simulink model "halfcontcon"  (R2021a)
settings: Solver=VariableStepAuto  StartTime=0.0  StopTime=5  FixedStep=1e-6  RelTol=1e-3
values from neighbouring files (symbols this model uses):
  Tr = (Pr*746)/(wr)    (= 20.3536435794)    [halfcontrolledconverter.m]
  vcontrol = cosd(alpha)    [halfcontrolledconverter.m]
  Vm = Vs_rms*(2)^(0.5)    (= 325.269119346)    [halfcontrolledconverter.m]
libraries: spsDiodeLib x6, spsVoltageMeasurementLib x3, spsCurrentMeasurementLib x2, simulink_extras x2, spsMonostableLib x2, spsThyristorLib x2, spsACVoltageSourceLib x1, spsDCMachineLib x1, spsGroundLib x1, spsSeriesRLCBranchLib x1, spspowerguiLib x1
settings Model: Creator=dinesh  LastModifiedBy=mluser
settings SolverCC: ZeroCrossAlgorithm=Adaptive  AlgebraicLoopSolver=TrustRegion
settings DataIOCC: ReturnWorkspaceOutputs=off
settings DebuggingCC: IgnoredZcDiagnostic=none  SFMachineParentedDataDiag=warning  ArithmeticOperatorsInVariantConditions=warning
settings SFSimCC: SimUseLocalCustomCode=off  CustomCodeUndefinedFunction=UseInterfaceOnly
settings RTWCC: RTWUseLocalCustomCode=off

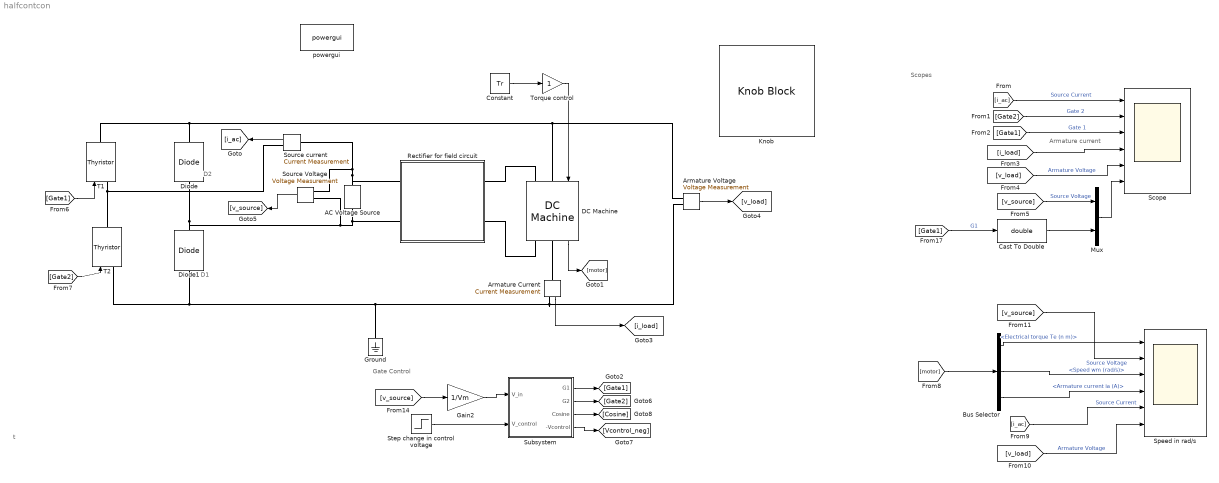
== system halfcontcon ==
  note: Armature current
  note: D2
  note: D1
  note: t
  note: Scopes
  note: Gate Control
  AC Voltage Source : spsACVoltageSourceLib/AC Voltage Source  Amplitude=Vm  Phase=0  Frequency=50  SampleTime=0  Measurements=None  BusType=swing  Pref=10e3  Qref=0  Qmin=-inf  Qmax=+inf
  Armature Current : spsCurrentMeasurementLib/Current Measurement  PhasorSimulation=off  OutputType=Complex  PSBequivalent=0
  Armature Voltage : spsVoltageMeasurementLib/Voltage Measurement  PhasorSimulation=off  OutputType=Complex  PSBequivalent=0
  Bus Selector : BusSelector  OutputSignals=Electrical torque Te (n m),Speed wm (rad/s),Armature current ia (A)
  Cast To Double : DataTypeConversion  OutDataTypeStr=double
  Constant : Constant  Value=Tr
  DC Machine : spsDCMachineLib/DC Machine  PresetModel=01: 5HP 240V 1750RPM Field:300V  MechanicalLoad=Torque TL  FieldType=Wound  ShowDetailedParameters=on  MeasurementBus=off  RLa=[2.581 0.028]  RLf=[281.2 156]  Laf=0.9483  MachineConstant=Torque constant (N.m/A)  Ke=1.8  Kt=1.8  J=0.02215  Bm=0.002953  Tf=0.5161  w0=1  Ifinit=0  TsPowergui=0  TsBlock=-1
  Diode : spsDiodeLib/Diode  Ron=0.001  Lon=0  Vf=0.8  IC=0  UseSnubber=0  Rs=inf  Cs=inf  Measurements=off
  Diode1 : spsDiodeLib/Diode  Ron=0.001  Lon=0  Vf=0.8  IC=0  UseSnubber=0  Rs=inf  Cs=inf  Measurements=off
  Gain2 : Gain  Gain=1/Vm
  Ground : spsGroundLib/Ground  LConnTagsString=a
  Knob : KnobBlock  LabelPosition=Bottom  ScaleMax=1
  Mux : Mux  Inputs=2
  Rectifier for field circuit : Subsystem
  Scope : Scope  NumInputPorts=6
  Source Voltage : spsVoltageMeasurementLib/Voltage Measurement  PhasorSimulation=off  OutputType=Complex  PSBequivalent=0
  Source current : spsCurrentMeasurementLib/Current Measurement  PhasorSimulation=off  OutputType=Complex  PSBequivalent=0
  Speed in rad/s : Scope  NumInputPorts=6
  Step change in control voltage : Step  Time=0  Before=0.1  After=vcontrol  SampleTime=0
  Subsystem : Subsystem
  T1 : spsThyristorLib/Thyristor  Ron=0.001  Lon=0  Vf=0.8  IC=0  Rs=inf  Cs=0.22e-6  Measurements=off
  T2 : spsThyristorLib/Thyristor  Ron=0.001  Lon=0  Vf=0.8  IC=0  Rs=inf  Cs=0.22e-6  Measurements=off
  Torque control : Gain
  powergui : spspowerguiLib/powergui  Priority=1  SimulationMode=Continuous  SampleTime=50e-6  frequency=60  Iterations=50  frequencyindice=0  Pbase=100e6  ErrMax=1e-4  UnitsV=kV  UnitsW=MW  buscounter=0  FunctionMessages=off  echomessages=off  EnableUseOfTLC=off  CurrentSourceSwitches=off  DisableSnubberDevices=off  DisableRonSwitches=off  DisableVfSwitches=off  DisplayEquations=off  AutomaticDiscreteSolvers=off  SolverType=Tustin/Backward Euler (TBE)  Interpol=off  ExternalGateDelay=off  methode=off  Ts=100  x0status=blocks  SPID=off  SwTol=0  HookPort=off  NonlinearTolerance=1e-4  nMaxIteration=100  ContinueOnMaxIteration=off  RestoreLinks=warning  ResistiveCurrentMeasurement=off  Frange=[0:2:500]  Ylog=off  Xlog=on  ShowGrid=off  save=off  variable=ZData  structure=0  ZoomFFT=off  StartTime=0.0  cycles=1  DisplayStyle=1  fundamental=60  FreqAxis=off  MaxFrequency=1000  frequencyindicesteady=1  RmsSteady=1  display=off
  wires:
  Source current/1 -> [i_ac]
  Armature Voltage/1 -> [v_load]
  Source Voltage/1 -> [v_source]
  [Gate1] -> T1/1
  [v_source] -> Gain2/1
  Subsystem/1(G1) -> [Gate1]
  Gain2/1 -> Subsystem/1(V_in)
  Subsystem/2(G2) -> [Gate2]
  Subsystem/3(Cosine) -> [Cosine]
  Subsystem/4(-Vcontrol) -> [Vcontrol_neg]
  [v_load] -> Scope/5  "Armature Voltage"
  [Gate1] -> Scope/3  "Gate 1"
  [i_ac] -> Scope/1  "Source Current"
  [i_load] -> Scope/4
  [v_source] -> Mux/1  "Source Voltage"
  Mux/1 -> Scope/6
  [Gate1] -> Cast To Double/1  "G1"
  Cast To Double/1 -> Mux/2
  Step change in control voltage/1 -> Subsystem/2(V_control)
  Bus Selector/1 -> Speed in rad/s/1  "<Electrical torque Te (n m)>"
  Bus Selector/2 -> Speed in rad/s/3  "<Speed wm (rad/s)>"
  [Gate2] -> T2/1
  Armature Current/1 -> [i_load]
  DC Machine/1 -> [motor]
  [motor] -> Bus Selector/1
  Constant/1 -> Torque control/1
  Torque control/1 -> DC Machine/1
  [Gate2] -> Scope/2  "Gate 2"
  Bus Selector/3 -> Speed in rad/s/4  "<Armature current ia (A)>"
  [i_ac] -> Speed in rad/s/5  "Source Current"
  [v_load] -> Speed in rad/s/6  "Armature Voltage"
  [v_source] -> Speed in rad/s/2  "Source Voltage"
  connections:
  AC Voltage Source/RConn1 -- Source current/LConn1 -- Source Voltage/LConn1 -- Rectifier for field circuit/RConn1
  Source current/RConn1 -- T2/RConn1 -- T1/LConn1
  Armature Current/RConn1 -- T2/LConn1 -- Diode1/LConn1 -- Ground/LConn1 -- Armature Voltage/LConn2
  AC Voltage Source/LConn1 -- Source Voltage/LConn2 -- Diode/LConn1 -- Diode1/RConn1 -- Rectifier for field circuit/RConn2
  T1/RConn1 -- DC Machine/LConn1 -- Armature Voltage/LConn1 -- Diode/RConn1
  Armature Current/LConn1 -- DC Machine/RConn1
  DC Machine/LConn2 -- Rectifier for field circuit/LConn1
  DC Machine/RConn2 -- Rectifier for field circuit/LConn2

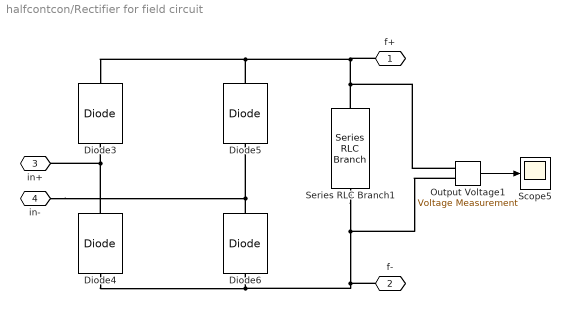
== system halfcontcon/Rectifier for field circuit ==
  Diode{3..6} (4 alike) : spsDiodeLib/Diode  Ron=0.001  Lon=0  Vf=0.8  IC=0  UseSnubber=0  Rs=inf  Cs=inf  Measurements=off
  Output Voltage1 : spsVoltageMeasurementLib/Voltage Measurement  PhasorSimulation=off  OutputType=Complex  PSBequivalent=0
  Scope5 : Scope
  Series RLC Branch1 : spsSeriesRLCBranchLib/Series RLC Branch  LConnTagsString=__new0  RConnTagsString=__new0  BranchType=C  Resistance=1  Inductance=1e-3  SetiL0=off  InitialCurrent=0  Capacitance=10e-3  Setx0=off  InitialVoltage=0  Measurements=None
  f+ : PMIOPort  Side=Left
  f- : PMIOPort  Port=2  Side=Left
  in+ : PMIOPort  Port=3  Side=Right
  in- : PMIOPort  Port=4  Side=Right
  wires:
  Output Voltage1/1 -> Scope5/1
  connections:
  Diode6/RConn1 -- in-/RConn1 -- Diode5/LConn1
  Diode4/RConn1 -- in+/RConn1 -- Diode3/LConn1
  Diode5/RConn1 -- Output Voltage1/LConn1 -- Series RLC Branch1/LConn1 -- f+/RConn1 -- Diode3/RConn1
  Diode4/LConn1 -- f-/RConn1 -- Series RLC Branch1/RConn1 -- Output Voltage1/LConn2 -- Diode6/LConn1

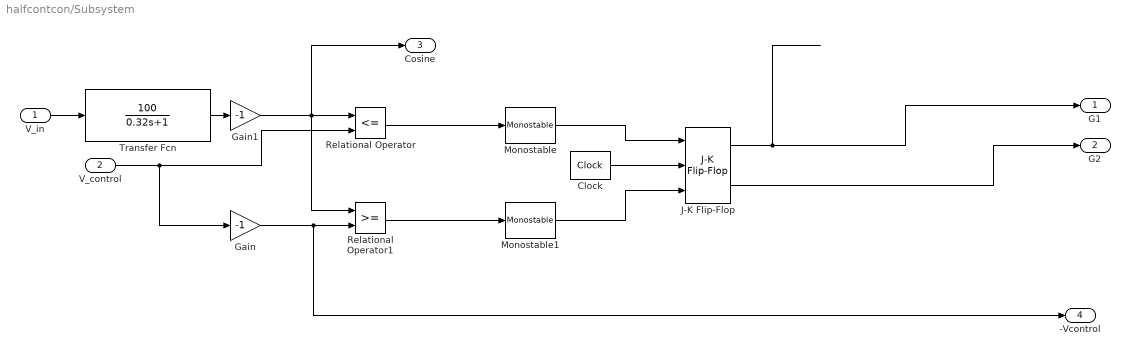
== system halfcontcon/Subsystem ==
  V_in : Inport
  V_control : Inport  Port=2
  Clock : simulink_extras/Flip Flops/Clock  period=100e-6
  Gain : Gain  Gain=-1
  Gain1 : Gain  Gain=-1
  J-K Flip-Flop : simulink_extras/Flip Flops/J-K Flip-Flop  initial_condition=0
  Monostable : spsMonostableLib/Monostable  EdgeDetect=Rising  PulseDuration=1e-3  ic=0  Ts=0
      settings: SourceProductBaseCode=PS
  Monostable1 : spsMonostableLib/Monostable  EdgeDetect=Rising  PulseDuration=1e-3  ic=0  Ts=0
      settings: SourceProductBaseCode=PS
  Relational Operator : RelationalOperator  Operator=<=  OutDataTypeStr=boolean  RndMeth=Simplest
  Relational Operator1 : RelationalOperator  OutDataTypeStr=boolean  RndMeth=Simplest
  Transfer Fcn : TransferFcn  Numerator=[100]  Denominator=[0.32 1]
  G1 : Outport  VectorParamsAs1DForOutWhenUnconnected=off
  G2 : Outport  Port=2  VectorParamsAs1DForOutWhenUnconnected=off
  Cosine : Outport  Port=3  VectorParamsAs1DForOutWhenUnconnected=off
  -Vcontrol : Outport  Port=4  VectorParamsAs1DForOutWhenUnconnected=off
  wires:
  Transfer Fcn/1 -> Gain1/1
  V_control/1 -> Relational Operator/2, Gain/1
  Gain/1 -> -Vcontrol/1, Relational Operator1/2
  Relational Operator/1 -> Monostable/1
  Relational Operator1/1 -> Monostable1/1
  V_in/1 -> Transfer Fcn/1
  Monostable/1 -> J-K Flip-Flop/1
  Monostable1/1 -> J-K Flip-Flop/3
  J-K Flip-Flop/1 -> G1/1
  J-K Flip-Flop/2 -> G2/1
  Clock/1 -> J-K Flip-Flop/2
  Gain1/1 -> Cosine/1, Relational Operator/1, Relational Operator1/1
